simulink subsystem "VITALINVERSEDPENDULUM"  (R2023a)
settings: Solver=VariableStepAuto  StartTime=0.0  StopTime=10.0  RelTol=1e-3
values from neighbouring files (symbols this model uses):
  g = 9.8    [constants.m]
  J = m * l^2 / 3    (= 0.0333333333333)    [constants.m]
  l = 1    [constants.m]
  m = .1    (= 0.1)    [constants.m]
  M = .2    (= 0.2)    [constants.m]
settings Model: Creator=ycheb  LastModifiedBy=ycheb

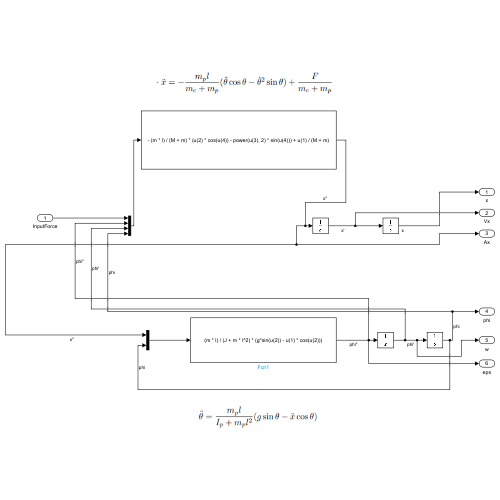
[thumbnail: Simulink's stored preview of the top-level diagram]
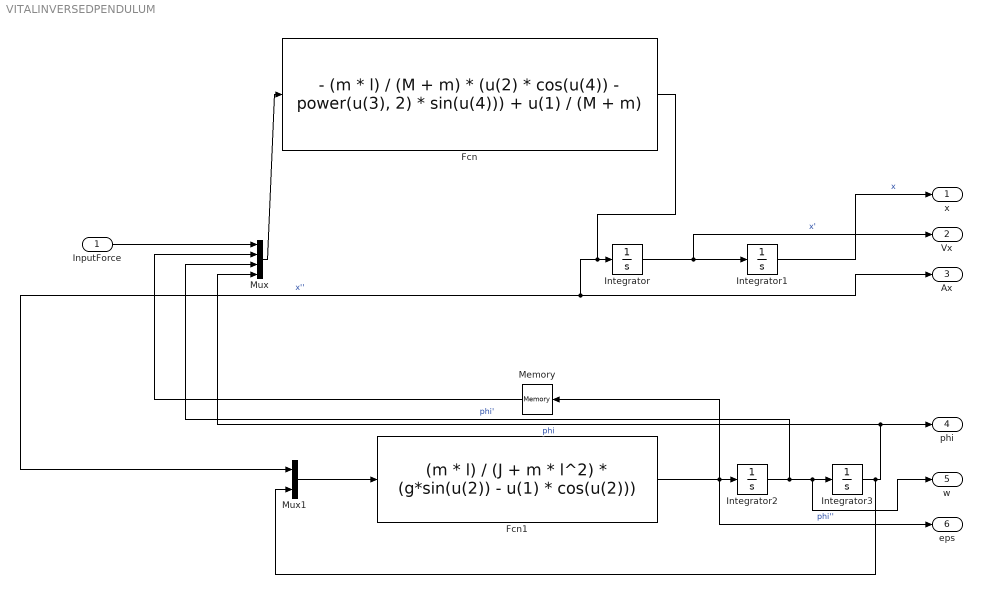
== system VITALINVERSEDPENDULUM ==
  InputForce : Inport
  Fcn : Fcn  Expr=- (m * l) / (M + m) * (u(2) * cos(u(4)) - power(u(3), 2) * sin(u(4))) + u(1) / (M + m)
  Fcn1 : Fcn  Expr=(m * l) / (J + m * l^2) * (g*sin(u(2)) - u(1) * cos(u(2)))
  Integrator : Integrator
  Integrator1 : Integrator
  Integrator2 : Integrator
  Integrator3 : Integrator  InitialCondition=-5 * pi / 180
  Memory : Memory
  Mux : Mux
  Mux1 : Mux  Inputs=2
  x : Outport
  Vx : Outport  Port=2
  Ax : Outport  Port=3
  phi : Outport  Port=4
  w : Outport  Port=5
  eps : Outport  Port=6
  wires:
  InputForce/1 -> Mux/1
  Mux/1 -> Fcn/1
  Fcn/1 -> Ax/1, Mux1/1, Integrator/1  "x''"
  Integrator/1 -> Vx/1, Integrator1/1  "x'"
  Mux1/1 -> Fcn1/1
  Fcn1/1 -> Memory/1, eps/1, Integrator2/1  "phi''"
  Integrator2/1 -> w/1, Integrator3/1, Mux/3  "phi'"
  Integrator3/1 -> Mux1/2, Mux/4, phi/1  "phi"
  Integrator1/1 -> x/1  "x"
  Memory/1 -> Mux/2
